simulink model "Shin_com"  (R2024a)
settings: Solver=VariableStepAuto  StartTime=0.0  StopTime=10.0  RelTol=1e-3
undefined symbols (not defined in the file): route1_waypoint_x, route1_waypoint_y, route2_waypoint_x, route2_waypoint_y, route3_waypoint_x, route3_waypoint_y, route4_waypoint_x, route4_waypoint_y, route5_waypoint_x, route5_waypoint_y
libraries: CarMaker4SL x162, slpidlib x4, robotalgslib x1, matrix_library x1
(part 4 of 4)

== matlab function Shin_com/Triggered Subsystem2/Function-Call Subsystem/MATLAB Function4 ==
  data: start input; goal input; obstacle_list input; full_path output
function full_path = main_rrt_rs(start, goal, obstacle_list) %#codegen

    space = [0, 100, -100, 0];
    max_iter = 3000; step_size = 1; goal_sample_rate = 0.4; radius = 10; R = 7;
    MAX_NODES = 3000;
    default_node = struct('pos', zeros(1,3), 'parent', int32(0), 'cost', Inf);
    nodes = repmat(default_node, 1, MAX_NODES);
    nodes(1).pos = start(:)';
    nodes(1).parent = int32(0);
    nodes(1).cost = 0.0;
    node_count = int32(1);
    goal = reshape(goal, 1, 3);
    start = reshape(start, 1, 3);

    c_best = inf; best_goal_node = int32(-1);
    rs_to_goal = NaN(200,3); rs_count = int32(0);

    for iter = 1:max_iter
        if rand < goal_sample_rate
            sample = goal;
        elseif isfinite(c_best)
            sample = informed_sample(start, goal, c_best, space);
        else
            sample = [ ...
                rand_range(space(1), space(2)), ...
                rand_range(space(3), space(4)), ...
                rand * 2 * pi ...
                ];
        end
        sample = reshape(sample, 1, 3);  % ✅ 안전성 확보
        min_dist = inf;
        nearest_id = int32(1);
        for i = 1:node_count
            d = norm(nodes(i).pos(1:2) - sample(1:2));
            if d < min_dist
                min_dist = d;
                nearest_id = int32(i);
            end
        end
        nearest_node = nodes(nearest_id);

        theta = atan2(sample(2) - nearest_node.pos(2), sample(1) - nearest_node.pos(1));
        new_pos = [nearest_node.pos(1:2) + step_size * [cos(theta), sin(theta)], theta];

        if ~collision_check_line(nearest_node.pos, new_pos, obstacle_list, space)
            new_node = struct('pos', new_pos, ...
                'parent', int32(nearest_id), ...
                'cost', nearest_node.cost + norm(new_pos(1:2) - nearest_node.pos(1:2)));

            for i = 1:node_count
                if norm(nodes(i).pos(1:2) - new_node.pos(1:2)) < radius
                    temp_cost = nodes(i).cost + norm(nodes(i).pos(1:2) - new_node.pos(1:2));
                    if temp_cost < new_node.cost && ~collision_check_line(nodes(i).pos, new_node.pos, obstacle_list, space)
                        new_node.cost = temp_cost;
                        new_node.parent = int32(i);
                    end
                end
            end

            if node_count < MAX_NODES
                node_count = node_count + 1;
                nodes(node_count) = new_node;
            end

            if norm(new_node.pos(1:2) - goal(1:2)) < 25
                [valid, rs_path] = reeds_shepp_connect(new_node.pos, goal, R, obstacle_list, space);
                if valid
                    c_rs = new_node.cost + compute_rs_cost(rs_path);
                    if c_rs < c_best
                        c_best = c_rs;
                        best_goal_node = node_count;
                        rs_count = int32(min(size(rs_path,1), size(rs_to_goal,1)));
                        rs_to_goal(1:rs_count,:) = rs_path(1:rs_count,:);
                    end
                end
            end
        end
    end

    if best_goal_node > 0
        path_temp = zeros(300, 3);
        count = int32(0);
        current = best_goal_node;
        while current > 0
            count = count + 1;
            path_temp(count,:) = nodes(current).pos;
            current = nodes(current).parent;
        end
        rrt_path = flipud(path_temp(1:count,:));
        rrt_path = path_clothoid_smoothing(rrt_path); % 고급 smoothing 적용
        n_rrt = size(rrt_path,1);
        full_path = NaN(300,3);
        full_path(1:n_rrt,:) = rrt_path;
        full_path(n_rrt+1:n_rrt+rs_count,:) = rs_to_goal(1:rs_count,:);
    else
        full_path = NaN(300,3);
    end
    function r = rand_range(a, b) %#codegen
        r = a + (b - a) * rand;
    end
end
function sample = informed_sample(start, goal, c_max, space) %#codegen
    % === 고정된 출력: 반드시 [1×3] 벡터 ===
    sample = zeros(1, 3);

    % === 타원 파라미터 계산 ===
    c_min = norm(goal(1:2) - start(1:2));
    a = c_max / 2;
    b = sqrt(max(1e-6, c_max^2 - c_min^2)) / 2;
    theta = atan2(goal(2) - start(2), goal(1) - start(1));
    cos_t = cos(theta);
    sin_t = sin(theta);
    mid = 0.5 * (start(1:2) + goal(1:2));

    % === 고정 반복 횟수 시도 (예: 50회) ===
    for i = 1:50
        x = a * (2 * rand - 1);  % [-a, a]
        y = b * (2 * rand - 1);  % [-b, b]

        % 타원 내부 점만 사용
        if (x^2 / a^2 + y^2 / b^2) <= 1
            pos_x = cos_t * x - sin_t * y + mid(1);
            pos_y = sin_t * x + cos_t * y + mid(2);
            yaw   = 2 * pi * rand;

            sample(1) = pos_x;
            sample(2) = pos_y;
            sample(3) = yaw;
            return;
        end
    end

    % 실패 시 fallback: goal 반환
    sample = goal(:)';  % [1×3] 형태 유지
end

function smooth_path = path_clothoid_smoothing(path)
    if size(path, 1) < 3
        smooth_path = path;
        return;
    end

    fixed_points = false(size(path, 1), 1);
    for i = 2:size(path, 1) - 1
        prev = path(i - 1, 1:2);
        curr = path(i, 1:2);
        next = path(i + 1, 1:2);
        angle1 = atan2(curr(2) - prev(2), curr(1) - prev(1));
        angle2 = atan2(next(2) - curr(2), next(1) - curr(1));
        if abs(angle1 - angle2) < deg2rad(5)
            fixed_points(i) = true;
        end
    end

    x = path(:, 1); y = path(:, 2); yaw = path(:, 3);
    s = cumsum([0; sqrt(diff(x).^2 + diff(y).^2)]);
    ts = linspace(0, s(end), 5 * numel(s));
    x_smooth = interp1(s(~fixed_points), x(~fixed_points), ts, 'pchip', 'extrap');
    y_smooth = interp1(s(~fixed_points), y(~fixed_points), ts, 'pchip', 'extrap');
    yaw_unwrap = unwrap(yaw);
    yaw_smooth = interp1(s(~fixed_points), yaw_unwrap(~fixed_points), ts, 'pchip', 'extrap');

    dx = gradient(x_smooth); dy = gradient(y_smooth);
    ddx = gradient(dx); ddy = gradient(dy);
    curvature = abs((dx .* ddy - dy .* ddx) ./ (dx.^2 + dy.^2).^(3/2));
    max_curvature = 0.05;

    for k = 2:length(curvature)
        if curvature(k) > max_curvature
            factor = max_curvature / curvature(k);
            x_smooth(k) = x_smooth(k-1) + factor * (x_smooth(k) - x_smooth(k-1));
            y_smooth(k) = y_smooth(k-1) + factor * (y_smooth(k) - y_smooth(k-1));
        end
    end
    smooth_path = [x_smooth',...
                    y_smooth',...
                    wrapToPi(yaw_smooth')];
end

function [valid, rs_path] = reeds_shepp_connect(start, goal, R, obstacle_list, space)
    param.step = 0.5;
    param.max_curv = 1 / R;
    [x_list, y_list, yaw_list] = generation(start, goal, param);
    rs_path = [x_list(:), y_list(:), yaw_list(:)];
    valid = true;
    for i = 1:size(rs_path,1)
        pos = rs_path(i, :);
        if collision_check_point(pos, obstacle_list, space)
            valid = false;
            return;
        end
    end
end

function cost = compute_rs_cost(rs_path)
    % rs_path: [N x 3] 형태의 Reeds-Shepp 경로 (x, y, yaw)
    % 두 점 사이의 유클리디안 거리 누적합을 사용한 비용 계산
    if size(rs_path,1) < 2
        cost = 0;
        return;
    end
    dx = diff(rs_path(:,1));
    dy = diff(rs_path(:,2));
    dist = hypot(dx, dy);
    cost = sum(dist);
end

function is_collision = collision_check_line(start_pos, end_pos, obstacle_list, space) %#codegen
    % 간단한 선분-장애물 교차 검사: 샘플링 방식 사용
    n = 10;
    is_collision = false;
    for i = 0:n
        t = i / n;
        pos = (1 - t) * start_pos + t * end_pos;
        if collision_check_point(pos, obstacle_list, space)
            is_collision = true;
            return;
        end
    end
end

function is_collision = collision_check_point(pos, obstacle_list, space)
    x = pos(1); y = pos(2);
    if x < space(1) || x > space(2) || y < space(3) || y > space(4)
        is_collision = true;
        return;
    end
    is_collision = false;
    for i = 1:size(obstacle_list, 1)
        dx = x - obstacle_list(i,1);
        dy = y - obstacle_list(i,2);
        if hypot(dx, dy) < obstacle_list(i,3) + 1.5
            is_collision = true;
            return;
        end
    end
end

function [x_list, y_list, yaw_list] = generation(start_pose, goal_pose, param)
    sx = start_pose(1); sy = start_pose(2); syaw = start_pose(3);
    gx = goal_pose(1); gy = goal_pose(2); gyaw = goal_pose(3);

    dx = gx - sx; dy = gy - sy; dyaw = gyaw - syaw;
    x = (cos(syaw) * dx + sin(syaw) * dy) * param.max_curv;
    y = (-sin(syaw) * dx + cos(syaw) * dy) * param.max_curv;
    planner_fns = {@SCS, @CCC, @CSC, @CCCC, @CCSC};

    best_cost = inf;
    best_path = struct('segs', zeros(1,3), 'ctypes', ['L','S','L'], 'len', inf);

    % === 3) 각 플래너로부터 후보 경로 받아 최저 비용 갱신 ===
    for pi = 1:numel(planner_fns)
        paths = planner_fns{pi}(x, y, dyaw);
        for k = 1:numel(paths)
            if paths(k).len < best_cost
                best_cost = paths(k).len;
                best_path = paths(k);
            end
        end
    end

    % === 4) 유효한 경로가 하나도 없으면 빈 배열 리턴(선택사항) ===
    if isinf(best_cost)
        x_list = zeros(0,1); 
        y_list = zeros(0,1); 
        yaw_list = zeros(0,1);
        return;
    end

    points_num = floor(best_cost / param.step) + length(best_path.segs) + 5;
    x_list_ = zeros(points_num, 1);
    y_list_ = zeros(points_num, 1);
    yaw_list_ = zeros(points_num, 1);

    i = 1;
    x = 0; y = 0; yaw = 0;
    for j = 1:length(best_path.segs)
        m = best_path.ctypes(j);
        seg_length = best_path.segs(j);
        if seg_length == 0
            continue;   % 0 길이 세그먼트는 건너뛸 것
        end
        d_length = param.step * sign(seg_length);
        l = 0;
        while abs(l) <= abs(seg_length)
            new_pt = interpolate(m, l, [x, y, yaw], param);
            i = i + 1;
            x_list_(i) = new_pt(1);
            y_list_(i) = new_pt(2);
            yaw_list_(i) = new_pt(3);
            l = l + d_length;
        end
        new_pt = interpolate(m, seg_length, [x, y, yaw], param);
        i = i + 1;
        x_list_(i) = new_pt(1);
        y_list_(i) = new_pt(2);
        yaw_list_(i) = new_pt(3);
        x = new_pt(1); y = new_pt(2); yaw = new_pt(3);
    end

    x_list_ = x_list_(1:i);
    y_list_ = y_list_(1:i);
    yaw_list_ = yaw_list_(1:i);

    x_list = zeros(size(x_list_));
    y_list = zeros(size(y_list_));
    yaw_list = zeros(size(yaw_list_));
    for k = 1:length(x_list_)
        x_list(k) = cos(-syaw) * x_list_(k) + sin(-syaw) * y_list_(k) + sx;
        y_list(k) = -sin(-syaw) * x_list_(k) + cos(-syaw) * y_list_(k) + sy;
        yaw_list(k) = M(yaw_list_(k) + syaw);
    end
end

function [r, theta] = R(x, y)
    r = hypot(x, y);
    theta = atan2(y, x);
end

function theta_truncate = M(theta)
    while theta > pi
        theta = theta - 2.0 * pi;
    end
    while theta < -pi
        theta = theta + 2.0 * pi;
    end
    theta_truncate = theta;
end

function [tau, omega] = calTauOmega(u, v, xi, eta, phi)
    delta = M(u - v);
    A = sin(u) - sin(delta);
    B = cos(u) - cos(delta) - 1.0;

    t1 = atan2(eta * A - xi * B, xi * A + eta * B);
    t2 = 2.0 * (cos(delta) - cos(v) - cos(u)) + 3.0;

    if t2 < 0
        tau = M(t1 + pi);
    else
        tau = M(t1);
    end
    omega = M(tau - u + v - phi);
end
function segs = SLS(x, y, phi)
    % Straight-Left-Straight generation mode.
    segs = [];
    
    phi = M(phi);
    if y > 0.0 && phi > 0.0 && phi < pi * 0.99
        xd = -y / tan(phi) + x;
        t = xd - tan(phi / 2.0);
        u = phi;
        v = hypot(x - xd, y) - tan(phi / 2.0);
        segs = [t, u, v];
    elseif y < 0.0 && phi > 0.0 && phi < pi * 0.99
        xd = -y / tan(phi) + x;
        t = xd - tan(phi / 2.0);
        u = phi;
        v = -hypot(x - xd, y) - tan(phi / 2.0);
        segs = [t, u, v];
    end
end

function segs = LRL(x, y, phi)
    % Left-Right-Left generation mode. (L+R-L-)
    segs = [];
    [r, theta] = R(x - sin(phi), y - 1.0 + cos(phi));
    if r <= 4.0
        u = -2.0 * asin(0.25 * r);
        t = M(theta + 0.5 * u + pi);
        v = M(phi - t + u);
        if t >= 0.0 && u <= 0.0
            segs = [t, u, v];
        end
    end
end

function segs = LSL(x, y, phi)
    % Left-Straight-Left generation mode. (L+S+L+)
    segs = [];
    
    [u, t] = R(x - sin(phi), y - 1.0 + cos(phi));
    if t >= 0.0
        v = M(phi - t);
        if v >= 0.0
            segs = [t, u, v];
        end
    end
end

function segs = LSR(x, y, phi)
    % Left-Straight-Right generation mode. (L+S+R+)
    segs = [];
    
    [r, theta] = R(x + sin(phi), y - 1.0 - cos(phi));
    r = r * r;
    if r >= 4.0
        u = sqrt(r - 4.0);
        t = M(theta + atan2(2.0, u));
        v = M(t - phi);
        if t >= 0.0 && v >= 0.0
            segs = [t, u, v];
        end
    end
end

function segs = LRLRn(x, y, phi)
    % Left-Right(beta)-Left(beta)-Right generation mode. (L+R+L-R-)
    segs = [];
    
    xi = x + sin(phi);
    eta = y - 1.0 - cos(phi);
    rho = 0.25 * (2.0 + hypot(xi, eta));
    if rho <= 1.0
        u = acos(rho);
        [t, v] = calTauOmega(u, -u, xi, eta, phi);
        if t >= 0.0 && v <= 0.0
            segs = [t, u, v];
        end
    end
end

function segs = LRLRp(x, y, phi)
    % Left-Right(beta)-Left(beta)-Right generation mode. (L+R-L-R+)
    segs = [];
    
    xi = x + sin(phi);
    eta = y - 1.0 - cos(phi);
    rho = (20.0 - xi * xi - eta * eta) / 16.0;
    if 0.0 <= rho && rho <= 1.0
        u = -acos(rho);
        if u >= -0.5 * pi
            [t, v] = calTauOmega(u, u, xi, eta, phi);
            if t >= 0.0 && v >= 0.0
                segs = [t, u, v];
            end
        end
    end
end

function segs = LRSR(x, y, phi)
    % Left-Right(pi/2)-Straight-Right generation mode. (L+R-S-R-)
    segs = [];
    
    xi = x + sin(phi);
    eta = y - 1.0 - cos(phi);
    [rho, theta] = R(-eta, xi);

    if rho >= 2.0
        t = theta;
        u = 2.0 - rho;
        v = M(t + 0.5 * pi - phi);
        if t >= 0.0 && u <= 0.0 && v <= 0.0
            segs = [t, u, v];
        end
    end
end

function segs = LRSL(x, y, phi)
    % Left-Right(pi/2)-Straight-Left generation mode. (L+R-S-L-)
    segs = [];
    
    xi = x - sin(phi);
    eta = y - 1.0 + cos(phi);
    [rho, theta] = R(xi, eta);
    if rho >= 2.0
        r = sqrt(rho * rho - 4.0);
        u = 2.0 - r;
        t = M(theta + atan2(r, -2.0));
        v = M(phi - 0.5 * pi - t);
        if t >= 0.0 && u <= 0.0 && v <= 0.0
            segs = [t, u, v];
        end
    end
end

function segs = LRSLR(x, y, phi)
    % Left-Right(pi/2)-Straight-Left(pi/2)-Right generation mode. (L+R-S-L-R+)
    segs = [];
    
    xi = x + sin(phi);
    eta = y - 1.0 - cos(phi);
    [r, ~] = R(xi, eta);
    if r >= 2.0
        u = 4.0 - sqrt(r * r - 4.0);
        if u <= 0.0
            t = M(atan2((4.0 - u) * xi - 2.0 * eta, -2.0 * xi + (u - 4.0) * eta));
            v = M(t - phi);
            if t >= 0.0 && v >= 0.0
                segs = [t, u, v];
            end
        end
    end
end

function path = RSPath(segs_in, ctypes_in)
    MAX_LEN = 5;  % 최대 5개 segment까지 허용
    segs_fixed = zeros(1, MAX_LEN);
    ctypes_fixed = repmat(' ', 1, MAX_LEN);

    n = length(segs_in);
    segs_fixed(1:n) = segs_in;

    for i = 1:n
        ctypes_fixed(i) = ctypes_in{i};
    end

    path.segs = segs_fixed;
    path.ctypes = ctypes_fixed;
    path.len = sum(abs(segs_in(:)));  % ✅ 항상 스칼라
end

    
function paths = SCS(x, y, phi) %#codegen
    MAX_PATHS = 2;
    paths = init_rs_paths(MAX_PATHS);
    cnt = uint8(0);

    segs = SLS(x, y, phi);
    if ~isempty(segs)
        cnt = cnt + 1;
        paths(cnt) = RSPath(segs, {'S', 'L', 'S'});
    end

    segs = SLS(x, -y, -phi);
    if ~isempty(segs)
        cnt = cnt + 1;
        paths(cnt) = RSPath(segs, {'S', 'R', 'S'});
    end

    paths = paths(1:cnt);
end

function paths = CCC(x, y, phi) %#codegen
    MAX_PATHS = 8;
    paths = init_rs_paths(MAX_PATHS);
    cnt = uint8(0);

    cases = {
        LRL(x, y, phi),            {'L','R','L'};
        -LRL(-x, y, -phi),         {'L','R','L'};
        LRL(x, -y, -phi),          {'R','L','R'};
        -LRL(-x, -y, phi),         {'R','L','R'};
    };

    for k = 1:size(cases,1)
        segs = cases{k,1};
        if ~isempty(segs)
            cnt = cnt + 1;
            paths(cnt) = RSPath(segs, cases{k,2});
        end
    end

    xb = x * cos(phi) + y * sin(phi);
    yb = x * sin(phi) - y * cos(phi);

    segs = LRL(xb, yb, phi);
    if ~isempty(segs)
        cnt = cnt + 1;
        paths(cnt) = RSPath([segs(3), segs(2), segs(1)], {'L','R','L'});
    end

    segs = LRL(-xb, yb, -phi);
    if ~isempty(segs)
        cnt = cnt + 1;
        paths(cnt) = RSPath(-[segs(3), segs(2), segs(1)], {'L','R','L'});
    end

    segs = LRL(xb, -yb, -phi);
    if ~isempty(segs)
        cnt = cnt + 1;
        paths(cnt) = RSPath([segs(3), segs(2), segs(1)], {'R','L','R'});
    end

    segs = LRL(-xb, -yb, phi);
    if ~isempty(segs)
        cnt = cnt + 1;
        paths(cnt) = RSPath(-[segs(3), segs(2), segs(1)], {'R','L','R'});
    end

    paths = paths(1:cnt);
end

function paths = CSC(x, y, phi) %#codegen
    MAX_PATHS = 8;
    paths = init_rs_paths(MAX_PATHS);
    cnt = uint8(0);

    segs_and_types = {
        LSL(x, y, phi),            {'L', 'S', 'L'};
        -LSL(-x, y, -phi),         {'L', 'S', 'L'};
        LSL(x, -y, -phi),          {'R', 'S', 'R'};
        -LSL(-x, -y, phi),         {'R', 'S', 'R'};
        LSR(x, y, phi),            {'L', 'S', 'R'};
        -LSR(-x, y, -phi),         {'L', 'S', 'R'};
        LSR(x, -y, -phi),          {'R', 'S', 'L'};
        -LSR(-x, -y, phi),         {'R', 'S', 'L'};
    };

    for k = 1:size(segs_and_types, 1)
        segs = segs_and_types{k,1};
        if ~isempty(segs)
            cnt = cnt + 1;
            paths(cnt) = RSPath(segs, segs_and_types{k,2});
        end
    end

    paths = paths(1:cnt);
end

function paths = CCCC(x, y, phi) %#codegen
    MAX_PATHS = 8;
    paths = init_rs_paths(MAX_PATHS);
    cnt = uint8(0);

    segs = LRLRn(x, y, phi);
    if ~isempty(segs)
        cnt = cnt + 1;
        paths(cnt) = RSPath([segs(1), segs(2), -segs(2), segs(3)], {'L','R','L','R'});
    end

    segs = LRLRn(-x, y, -phi);
    if ~isempty(segs)
        cnt = cnt + 1;
        paths(cnt) = RSPath([-segs(1), -segs(2), segs(2), -segs(3)], {'L','R','L','R'});
    end

    segs = LRLRn(x, -y, -phi);
    if ~isempty(segs)
        cnt = cnt + 1;
        paths(cnt) = RSPath([segs(1), segs(2), -segs(2), segs(3)], {'R','L','R','L'});
    end

    segs = LRLRn(-x, -y, phi);
    if ~isempty(segs)
        cnt = cnt + 1;
        paths(cnt) = RSPath([-segs(1), -segs(2), segs(2), -segs(3)], {'R','L','R','L'});
    end

    segs = LRLRp(x, y, phi);
    if ~isempty(segs)
        cnt = cnt + 1;
        paths(cnt) = RSPath([segs(1), segs(2), segs(2), segs(3)], {'L','R','L','R'});
    end

    segs = LRLRp(-x, y, -phi);
    if ~isempty(segs)
        cnt = cnt + 1;
        paths(cnt) = RSPath([-segs(1), -segs(2), -segs(2), -segs(3)], {'L','R','L','R'});
    end

    segs = LRLRp(x, -y, -phi);
    if ~isempty(segs)
        cnt = cnt + 1;
        paths(cnt) = RSPath([segs(1), segs(2), segs(2), segs(3)], {'R','L','R','L'});
    end

    segs = LRLRp(-x, -y, phi);
    if ~isempty(segs)
        cnt = cnt + 1;
        paths(cnt) = RSPath([-segs(1), -segs(2), -segs(2), -segs(3)], {'R','L','R','L'});
    end

    paths = paths(1:cnt);
end

function paths = CCSC(x, y, phi) %#codegen
    MAX_PATHS = 16;
    paths = init_rs_paths(MAX_PATHS);
    cnt = uint8(0);

    variants = {
        LRSL(x, y, phi),           {'L', 'R', 'S', 'L'}, [1 -0.5*pi 2 3];
        LRSL(-x, y, -phi),         {'L', 'R', 'S', 'L'}, [-1 0.5*pi -2 -3];
        LRSL(x, -y, -phi),         {'R', 'L', 'S', 'R'}, [1 -0.5*pi 2 3];
        LRSL(-x, -y, phi),         {'R', 'L', 'S', 'R'}, [-1 0.5*pi -2 -3];
        LRSR(x, y, phi),           {'L', 'R', 'S', 'R'}, [1 -0.5*pi 2 3];
        LRSR(-x, y, -phi),         {'L', 'R', 'S', 'R'}, [-1 0.5*pi -2 -3];
        LRSR(x, -y, -phi),         {'R', 'L', 'S', 'L'}, [1 -0.5*pi 2 3];
        LRSR(-x, -y, phi),         {'R', 'L', 'S', 'L'}, [-1 0.5*pi -2 -3];
    };

    for k = 1:size(variants,1)
        segs = variants{k,1};
        type = variants{k,2};
        idxs = variants{k,3};
        if ~isempty(segs)
            t = segs(abs(idxs(1))) * sign(idxs(1));
            u = segs(abs(idxs(3))) * sign(idxs(3));
            v = segs(abs(idxs(4))) * sign(idxs(4));
            paths(cnt + 1) = RSPath([t, idxs(2), u, v], type);
            cnt = cnt + 1;
        end
    end

    paths = paths(1:cnt);
end

function out = init_rs_paths(N)
    tmpl = struct('segs', zeros(1,5), 'ctypes', repmat(' ',1,5), 'len', 0);
    out = repmat(tmpl, N, 1);
end

function new_pt = interpolate(mode, length, init_pose, param)
    x = init_pose(1); y = init_pose(2); yaw = init_pose(3);

    if mode == 'S'
        new_x   = x + length / param.max_curv * cos(yaw);
        new_y   = y + length / param.max_curv * sin(yaw);
        new_yaw = yaw;
    elseif mode == 'L'
        new_x   = x + (sin(yaw + length) - sin(yaw)) / param.max_curv;
        new_y   = y - (cos(yaw + length) - cos(yaw)) / param.max_curv;
        new_yaw = yaw + length;
    elseif mode == 'R'
        new_x   = x - (sin(yaw - length) - sin(yaw)) / param.max_curv;
        new_y   = y + (cos(yaw - length) - cos(yaw)) / param.max_curv;
        new_yaw = yaw - length;
    else
        new_x = 0; new_y = 0; new_yaw = 0;
    end
    new_pt = [new_x, new_y, new_yaw];
end

== matlab function Shin_com/Triggered Subsystem2/Function-Call Subsystem1/MATLAB Function ==
  data: currPoseRear input; v input; waypoints input; delta output
function delta = lateral_spp_controller(currPoseRear, v, waypoints)
%▴ Hybrid Stanley & Pure Pursuit + Monotonic Index Enforcement
% Inputs:
%   currPoseRear : [x_rear; y_rear; psi] (후륜축 기준 위치 및 자세)
%   v            : 현재 속도 (m/s)
%   waypoints    : N×3 [x_i, y_i, psi_i] (경로 웨이포인트)
% Output:
%   delta        : 전륜 조향각 (rad)

    %#codegen
    %% persistent 변수 초기화
    persistent idx_last delta_prev
    if isempty(idx_last)
        idx_last   = 1;    % 마지막 타겟 인덱스 (초기값)
    end
    if isempty(delta_prev)
        delta_prev = 0;    % 이전 조향각 (로우패스 필터용)
    end

    %% 파라미터
    L        = 2.9;                             % 휠베이스 [m]
    k_st     = 1.0;                             % Stanley 이득
    eps_v    = 0.1;                             % 속도 안정화 상수
    deltaMax = deg2rad(40);                     % 최대 조향각 제한 ±40°
    e_thresh = 0.5;                             % SPP 전환 임계값 [m]
    k_pp     = 0.3;                             % 룩어헤드 속도 이득
    Ld_min   = 2.0;                             % 룩어헤드 최솟값 [m]
    Ld_max   = 4.0;                             % 룩어헤드 최댓값 [m]
    alpha_f  = 0.35;                            % 로우패스 필터 상수

    %% 전륜축 위치 계산 (후륜축 기준 → 전륜축 좌표 변환)
    x_f = currPoseRear(1) + L*cos(currPoseRear(3));
    y_f = currPoseRear(2) + L*sin(currPoseRear(3));

    %% 전방 웨이포인트만 선별 (로컬 좌표계)
    psi_wrapped = wrapToPi(currPoseRear(3));    % yaw를 –π~π로 유지
    heading_vec = [cos(psi_wrapped), sin(psi_wrapped)];
    diffs       = waypoints(:,1:2) - currPoseRear(1:2)';
    forward_idx = find(diffs * heading_vec' > 0);  % 전방 idx
    if isempty(forward_idx)
        forward_idx = (1:size(waypoints,1))';       % 전방이 없으면 전체 사용
    end

    %% 룩어헤드 거리 계산
    Ld_raw = k_pp * v + eps_v;
    Ld     = min(max(Ld_raw, Ld_min), Ld_max);

    %% 후보 인덱스 범위 설정 (룩어헤드 윈도우)
    N = size(waypoints,1);
    extra     = round(0.2 * Ld);                  % 윈도우 여분
    start_idx = max(idx_last - extra, 1);
    end_idx   = min(idx_last + round(Ld) + extra, N);
    cand_idx  = intersect(forward_idx, (start_idx:end_idx)');

    if isempty(cand_idx)
        cand_idx = forward_idx;  % 후보 없으면 전방 전체 사용
    end

    %% 최단거리 웨이포인트 선택
    dists = hypot(waypoints(cand_idx,1)-x_f, waypoints(cand_idx,2)-y_f);
    [~, rel] = min(dists);
    idx_new  = cand_idx(rel);  % 새로 계산된 인덱스

    %% 1) Monotonic Index Enforcement 적용
    % 새 인덱스(idx_new)가 이전 idx_last보다 작으면 무시
    if idx_new < idx_last
        idx_last = idx_last;    % 변경 없이 유지
    else
        idx_last = idx_new;     % 증가 시에만 갱신
    end

    %% 참조점 정보 추출
    x_ref   = waypoints(idx_last,1);
    y_ref   = waypoints(idx_last,2);
    psi_ref = waypoints(idx_last,3);

    %% Heading error 및 Cross-Track error 계산
    theta_e = wrapToPi(psi_ref - currPoseRear(3));  
    e_cte   = -(x_f - x_ref)*sin(psi_ref) + (y_f - y_ref)*cos(psi_ref);

    %% 제어 분기: Pure Pursuit vs Stanley
    if abs(e_cte) > e_thresh
        % Pure Pursuit
        alpha     = wrapToPi(atan2(y_ref-currPoseRear(2), x_ref-currPoseRear(1)) ...
                     - currPoseRear(3));
        delta_cmd = atan2(2 * L * sin(alpha), Ld);
    else
        % Stanley
        delta_cmd = theta_e + atan((k_st * e_cte) / (v + eps_v));
    end

    %% 로우패스 필터 적용 및 조향각 포화
    delta       = alpha_f * delta_cmd + (1 - alpha_f) * delta_prev;
    delta_prev  = delta;  
    delta       = max(min(delta, deltaMax), -deltaMax);

end

== matlab function Shin_com/Triggered Subsystem2/Function-Call Subsystem1/MATLAB Function2 ==
  settings: sampleTime=0.05
  data: currPoseRear input; DesiredAx output; ego_v input; target_velocity input; goalPose input; stopFlag output; target_velocity output
function [DesiredAx,stopFlag,target_velocity] = longitudinal_goal_controller(currPoseRear, ego_v,target_velocity,goalPose)
%▴ 종방향 속도 제어 및 목표 도달 확인
% Inputs:
%   currPoseRear: [x_rear; y_rear; psi] (후륜축 기준)
%   v           : 속도 (m/s)
%   goalPose    : [x_goal; y_goal; psi_goal]
% Outputs:
%   DesiredAx   : 원하는 가속도 (m/s^2)
%   stopFlag    : 목표 도달 시 true

    persistent Kp Kd dt prev_error
  if isempty(Kp)
    % — PD 게인 설정 (필요에 따라 조정하세요) —
    Kp = 1.8;    % 비례 이득
    Kd = 0.1;    % 미분 이득
    % — 제어 업데이트 주기 (Simulink 샘플타임과 동일하게) —
    dt = 0.1;    % [s]
    % — previous error 초기화 —
    prev_error = target_velocity - ego_v;
  end

  % 1) 속도 오차
  error = target_velocity - ego_v;
  % 2) 오차 변화율 (미분항)
  derivative = (error - prev_error) / dt;
  % 3) PD 제어 법칙
  DesiredAx = Kp * error + Kd * derivative;
  % 4) 이전 오차 갱신
  prev_error = error;


    %#codegen
    % 1) 위치·헤딩 오차 계산
    dx     = currPoseRear(1) - goalPose(1);
    dy     = currPoseRear(2) - goalPose(2);
    dist   = hypot(dx, dy);                                           % 거리 계산 :contentReference[oaicite:3]{index=3}
    yawErr = wrapToPi(goalPose(3) - currPoseRear(3));                 % –π~π 범위 :contentReference[oaicite:4]{index=4}

    % 2) 목표 도달 여부 판단 (Goal Checking in Parking Valet) :contentReference[oaicite:5]{index=5}
    posTol = 1.7;             % 위치 허용 오차 [m]
    yawTol = deg2rad(30);     % 헤딩 허용 오차 [rad]
    almostFlag = dist<12;
    distFlag = dist <= posTol;
    yawFlag = abs(yawErr) <= yawTol
    stopFlag = distFlag && yawFlag;

    % 3) DesiredAx 계산
    if stopFlag
        DesiredAx = -1000;
        disp("stopFlag")% 도착 시 완전 정지
    elseif almostFlag
        target_velocity = 3;
        disp("almost goal")% 근접 시 제동 가속도
        error      = target_velocity - ego_v;
        derivative = (error - prev_error)/dt;
        DesiredAx  = Kp*error + Kd*derivative;
        prev_error = error;
    end
end

== matlab function Shin_com/Triggered Subsystem2/Function-Call Subsystem1/MATLAB Function4 ==
  settings: sampleTime=0.05
  data: poly_coeff input; lateral_error output; velocity input; lookahead_time input; x_lookahead output
function [lateral_error, x_lookahead] = compute_lateral_error(poly_coeff, velocity, lookahead_time)
    
    % Lookahead 지점 계산
    x_lookahead = velocity * lookahead_time;
    % 경로 상의 lookahead 지점에서의 y값 계산
    y_desired = polyval(poly_coeff, x_lookahead);

    % lateral error : 차량 y=0 위치와 경로 y_desired의 차이
    lateral_error = y_desired;
end

== matlab function Shin_com/Triggered Subsystem2/Function-Call Subsystem1/MATLAB Function4  ==
  settings: sampleTime=0.05
  data: path input; local_waypoints_ output; vehicle_position input; head input
function local_waypoints_ = global_to_local_waypoints(path, vehicle_position, head)
    %#codegen
    % 글로벌 경로를 로컬 경로로 변환해주는 함수
    % path : [x, y, yaw] (경로 점들)
    % vehicle_position : [Ego_Global_X, Ego_Global_Y]
    % head : Ego_Yaw (rad)
    % 출력: 로컬 좌표 (x_local, y_local, yaw_local)

    % 최대 경로 점 개수 설정
    max_points = 100;

    % 초기화
    local_waypoints_ = NaN(max_points, 3);  % 고정 크기 배열

    % 차량 위치 및 헤딩 추출
    ego_x = vehicle_position(1);
    ego_y = vehicle_position(2);
    ego_yaw = head;

    % 회전 행렬 생성 (글로벌→로컬 변환)
    R = [cos(-ego_yaw) -sin(-ego_yaw); 
         sin(-ego_yaw)  cos(-ego_yaw)];

    count = int32(0);  % 경로 점 개수

    % 각 경로 포인트에 대해 변환 수행
    for i = 1:min(size(path, 1), max_points)
        % 글로벌 좌표에서 차량까지의 상대 위치
        dx = path(i, 1) - ego_x;  % X 좌표 차이
        dy = path(i, 2) - ego_y;  % Y 좌표 차이

        % 회전 변환 적용
        local_pos = R * [dx; dy];
        
        % Yaw 변환: 로컬 좌표계에서의 Yaw
        global_yaw = path(i, 3);
        local_yaw = wrapToPi(global_yaw - ego_yaw);  % 로컬 yaw 변환

        % 차량으로부터 waypoint까지의 거리
        distance = sqrt(local_pos(1)^2 + local_pos(2)^2);

        % 첫 번째 유효 경로 점 저장 (x > 0인 첫 포인트)
        if count == 0 && local_pos(1) > 0
            count = count + 1;
            local_waypoints_(count, :) = [local_pos(1), local_pos(2), local_yaw];
        end
        
        % 고정 크기 초과 방지
        if count < max_points
            count = count + 1;
            local_waypoints_(count, :) = [local_pos(1), local_pos(2), local_yaw];
        else
            warning('Maximum number of waypoints reached.');
            break;
        end
    end

    % 남은 부분을 NaN으로 채움
    if count < max_points
        local_waypoints_((count+1):max_points, :) = NaN;
    end
end

== matlab function Shin_com/Triggered Subsystem2/Function-Call Subsystem1/MATLAB Function5 ==
  settings: sampleTime=0.05
  data: local_waypoints input; poly_coeff output
function poly_coeff = fit_polynomial_to_waypoints(local_waypoints)
    % waypoint를 curve fitting 한 다항식 계수 반환
    % input: 로컬 좌표 웨이포인트
    % output: 다항식 계수 (3차)

    % 웨이포인트 추출
    x_points = local_waypoints(:, 1);  % 로컬 x 좌표
    y_points = local_waypoints(:, 2);  % 로컬 y 좌표

    % 유효한 웨이포인트만 사용 (x 좌표가 양수인 것만)
    valid_indices = x_points > 0;
    x_valid = x_points(valid_indices);
    y_valid = y_points(valid_indices);

    % 웨이포인트가 충분한지 확인
    if length(x_valid) < 4
        % 웨이포인트가 부족하면 직선 경로 반환
        poly_coeff = [0, 0, 0, 0];  % y = 0 (직선)
    else
        % 3차 다항식 피팅 (y = ax^3 + bx^2 + cx + d)
        poly_coeff = polyfit(x_valid, y_valid, 3);
    end
end

== matlab function Shin_com/Triggered Subsystem/MATLAB Function4 1 ==
  settings: sampleTime=0.05
  data: waypoint_x input; waypoint_y input; local_waypoints_ output; vehicle_position input; head input
function local_waypoints_ = global_to_local_waypoints(waypoint_x, waypoint_y, vehicle_position, head)

    % 초기화
    num_points = size(waypoint_x, 1);
    local_waypoints_ = NaN(num_points, 2);  % [x_local, y_local]

    % 차량 위치 추출
    ego_x = vehicle_position(1);
    ego_y = vehicle_position(2);
    ego_yaw = head;

    % 회전 행렬 생성 (글로벌→로컬 변환)
    R = [cos(-ego_yaw) -sin(-ego_yaw); 
         sin(-ego_yaw)  cos(-ego_yaw)];

    count = 0;
    % 각 웨이포인트에 대해 변환 수행
    for i = 1:num_points
        % 글로벌 좌표에서 차량까지의 상대 위치
        dx = waypoint_x(i) - ego_x;  % X 좌표 차이
        dy = waypoint_y(i) - ego_y;  % Y 좌표 차이

        % 회전 변환 적용
        local_pos = R * [dx; dy];
        distance = sqrt(dx.^2 + dy.^2); % 차량으로부터 waypoint까지의 길이 계산

        % 시작 좌표 저장
        if count == 0 && local_pos(1) > 0 && distance < 15
            count = count + 1;
            local_waypoints_(count, :) = [local_pos(1) local_pos(2)];     % 로컬 x 좌표 
        end

        % 아래의 조건을 모두 만족하는 경우에만 좌표 저장
        % 1. x 좌표가 0보다 큰 경우
        % 2. x의 현재 좌표가 이전 x의 좌표보다 큰 경우
        % 3. 차량으로부터 waypoint까지의 길이가 30m 이내인 경우 (길이는 임의로 테스트 한 후 설정 가능할 듯)
        if count  ~= 0 && local_pos(1) > 0 && local_pos(1) > local_waypoints_(count, 1)  && distance < 15
            count = count + 1;
            local_waypoints_(count, :) = [local_pos(1) local_pos(2)];
        end
    end
end

== matlab function Shin_com/Subsystem2/MATLAB Function4 ==
  settings: sampleTime=0.05
  data: poly_coeff input; lateral_error output; velocity input; lookahead_time input; x_lookahead output
function [lateral_error, x_lookahead] = compute_lateral_error(poly_coeff, velocity, lookahead_time)
    % Lookahead 지점 계산
    x_lookahead = velocity * lookahead_time + 2.9;

    % 경로 상의 lookahead 지점에서의 y값 계산
    y_desired = polyval(poly_coeff, x_lookahead);

    % lateral error : 차량 y=0 위치와 경로 y_desired의 차이
    lateral_error = y_desired;
end

== matlab function Shin_com/Subsystem2/MATLAB Function4  ==
  settings: sampleTime=0.05
  data: waypoints input; local_waypoints_ output; vehicle_position input; head input
function local_waypoints_ = global_to_local_waypoints(waypoints, vehicle_position, head)
    % 글로벌 좌표를 로컬 좌표로 변환해주는 함수
    % waypoints : Global_Waypoints [id, X, Y]
    % vehicle_position : [Ego_Global_X, Ego_Global_Y]
    % head : Ego_Yaw (rad)
    % 출력: Local Waypoints

    % 초기화
    num_points = size(waypoints, 1);
    local_waypoints_ = NaN(num_points, 2);  % [x_local, y_local]

    % 차량 위치 추출
    ego_x = vehicle_position(1);
    ego_y = vehicle_position(2);
    ego_yaw = head;

    % 회전 행렬 생성 (글로벌→로컬 변환)
    R = [cos(-ego_yaw) -sin(-ego_yaw); 
         sin(-ego_yaw)  cos(-ego_yaw)];

    count = 0;
    % 각 웨이포인트에 대해 변환 수행
    for i = 1:num_points
        % 글로벌 좌표에서 차량까지의 상대 위치
        dx = waypoints(i, 1) - ego_x;  % X 좌표 차이
        dy = waypoints(i, 2) - ego_y;  % Y 좌표 차이

        % 회전 변환 적용
        local_pos = R * [dx; dy];
        distance = sqrt(dx.^2 + dy.^2); % 차량으로부터 waypoint까지의 길이 계산

        % 시작 좌표 저장
        if count == 0 && local_pos(1) > 0 && distance < 15
            count = count + 1;
            local_waypoints_(count, :) = [local_pos(1) local_pos(2)];     % 로컬 x 좌표 
        end

        % 아래의 조건을 모두 만족하는 경우에만 좌표 저장
        % 1. x 좌표가 0보다 큰 경우
        % 2. x의 현재 좌표가 이전 x의 좌표보다 큰 경우
        % 3. 차량으로부터 waypoint까지의 길이가 30m 이내인 경우 (길이는 임의로 테스트 한 후 설정 가능할 듯)
        if count  ~= 0 && local_pos(1) > 0 && local_pos(1) > local_waypoints_(count, 1)  && distance < 15
            count = count + 1;
            local_waypoints_(count, :) = [local_pos(1) local_pos(2)];
        end
    end
end

== matlab function Shin_com/Subsystem2/MATLAB Function7 ==
  settings: sampleTime=0.05
  data: local_waypoints input; poly_coeff output
function poly_coeff = fit_polynomial_to_waypoints(local_waypoints)
    % waypoint를 curve fitting 한 다항식 계수 반환
    % input: 로컬 좌표 웨이포인트
    % output: 다항식 계수 (3차)

    % 웨이포인트 추출
    x_points = local_waypoints(:, 1);  % 로컬 x 좌표
    y_points = local_waypoints(:, 2);  % 로컬 y 좌표

    % 유효한 웨이포인트만 사용 (x 좌표가 양수인 것만)
    valid_indices = x_points > 0;
    x_valid = x_points(valid_indices);
    y_valid = y_points(valid_indices);
    poly_coeff = polyfit(x_valid, y_valid, 3);
end

== stateflow chart Shin_com/Triggered Subsystem2/Chart1 ==
  settings: sampleTime=0.05
  state drawMap
    entry:
    draw_Map();
  state goParking
    during:
    go_Parking();
  (default) -> drawMap
  drawMap -> goParking : after(10,tick)
  events: go_Parking output FUNCTION_CALL_EVENT; draw_Map output FUNCTION_CALL_EVENT

== matlab function Shin_com/Triggered Subsystem2/Function-Call Subsystem/MATLAB Function ==
  data: path input; ordered_path output
function ordered_path = reorder_path(path)
    %#codegen
    % 입력: path (100x3) - 역순 경로
    % 출력: ordered_path (100x3) - 정순 경로

    % 고정 크기 배열 선언 (100x3)
    ordered_path = NaN(300, 3);  
    
    % 유효 경로 필터링 (NaN 값 제거)
    valid_idx = ~isnan(path(:, 1)) & ~isnan(path(:, 2)) & ~isnan(path(:, 3));
    valid_path = path(valid_idx, :);

    % 유효 경로 개수
    num_points = size(valid_path, 1);

    % 역순으로 배열 채우기 (고정 크기 유지)
    for i = 1:num_points
        ordered_path(i, :) = valid_path(num_points - i + 1, :);
    end

    % 나머지 부분 NaN으로 채우기
    if num_points < 100
        ordered_path((num_points+1):100, :) = NaN;
    end
end

== matlab function Shin_com/Triggered Subsystem/MATLAB Function5 ==
  settings: sampleTime=0.05
  data: x input; x_best output; y input; v input; map_x input; y_best output; map_y input; x_all output; y_all output; obs_x input; obs_y input
function [x_best, y_best, x_all, y_all] = FrenetTrajectoryGenerator(x, y, v, map_x, map_y, obs_x, obs_y)
% 설정
DF_set = [-3.5, 0, 3.5];  % 차선 오프셋 후보 (좌, 중앙, 우)
K_J = 0.1; K_T = 0.1; K_D = 10.0; K_V = 1.0; K_LAT = 2.0; K_LON = 1.0;
target_speed = 15;
T = 1.0;
dt = 0.05;
ego_radius = 2.0;

M = length(DF_set);
N = round(T / dt);

x_all = zeros(N, M);
y_all = zeros(N, M);

% 장애물 정보
obs_r = 2.0;
num_obs = 8;

% 기준 경로 길이 계산
map_s = zeros(length(map_x), 1);
for i = 2:length(map_x)
    dx = map_x(i) - map_x(i-1);
    dy = map_y(i) - map_y(i-1);
    map_s(i) = map_s(i-1) + hypot(dx, dy);
end

% 현재 위치를 Frenet 좌표로 변환
[s0, d0] = getFrenet(x, y, map_x, map_y, map_s);
si = s0; si_d = v; si_dd = 0;
di = d0; di_d = 0; di_dd = 0;

costs = inf(1, M);  % 각 경로의 비용
trajectories = cell(M,2);  % x/y trajectory 저장

for k = 1:M
    d_target = DF_set(k);

    % Lateral (Quintic)
    a0 = di; a1 = di_d; a2 = 0.5 * di_dd;
    A_lat = [T^3 T^4 T^5; 3*T^2 4*T^3 5*T^4; 6*T 12*T^2 20*T^3];
    b_lat = [d_target - a0 - a1*T - a2*T^2; -a1 - 2*a2*T; -2*a2];
    coeff_d = A_lat \ b_lat;

    % Longitudinal (Quartic)
    b0 = si; b1 = si_d; b2 = 0.5 * si_dd;
    A_lon = [3*T^2 4*T^3; 6*T 12*T^2];
    b_lon = [target_speed - b1 - 2*b2*T; -2*b2];
    coeff_s = A_lon \ b_lon;

    s_traj = zeros(N,1); d_traj = zeros(N,1);
    x_traj = zeros(N,1); y_traj = zeros(N,1);
    jerk_d = 0; jerk_s = 0;
    is_collision = false;

    for i = 1:N
        t = (i-1)*dt;
        s_traj(i) = b0 + b1*t + b2*t^2 + coeff_s(1)*t^3 + coeff_s(2)*t^4;
        d_traj(i) = a0 + a1*t + a2*t^2 + coeff_d(1)*t^3 + coeff_d(2)*t^4 + coeff_d(3)*t^5;

        j_d = 6*coeff_d(1) + 24*coeff_d(2)*t + 60*coeff_d(3)*t^2;
        j_s = 6*coeff_s(1) + 24*coeff_s(2)*t;
        jerk_d = jerk_d + j_d^2;
        jerk_s = jerk_s + j_s^2;

        [xg, yg] = getCartesian(s_traj(i), d_traj(i), map_x, map_y, map_s);
        x_traj(i) = xg;
        y_traj(i) = yg;

        % 충돌 체크
        for j = 1:num_obs
            obs_dist = hypot(xg - obs_x(j), yg - obs_y(j));
            if obs_dist < (ego_radius + obs_r)
                is_collision = true;
            end
        end
    end

    x_all(:,k) = x_traj;
    y_all(:,k) = y_traj;

    if ~is_collision
        d_diff = (d_traj(end))^2;
        v_diff = (target_speed - (s_traj(end)-s_traj(1))/T)^2;
        cost_lat = K_J*jerk_d + K_T*T + K_D*d_diff;
        cost_lon = K_J*jerk_s + K_T*T + K_V*v_diff;
        costs(k) = K_LAT*cost_lat + K_LON*cost_lon;
    end

    trajectories{k,1} = x_traj;
    trajectories{k,2} = y_traj;
end

% === 유지 조건을 위한 persistent 변수들 ===
persistent prev_best_idx hold_count
if isempty(prev_best_idx)
    prev_best_idx = 2; % 초기엔 중앙 차선
    hold_count = 0;
end

% 최적 경로 선택
[best_cost, new_best_idx] = min(costs);

% 히스테리시스 조건
threshold = 5.0;                 % 얼마나 좋아야 바꿀지
hold_limit = 3.0 / dt;           % 유지 프레임 수 (3초)
current_cost = costs(prev_best_idx);

% 경로 변경 조건
if (new_best_idx ~= prev_best_idx) && ...
        (best_cost + threshold < current_cost || hold_count >= hold_limit)
    % 변경 허용
    prev_best_idx = new_best_idx;
    hold_count = 0;
else
    % 경로 유지
    new_best_idx = prev_best_idx;
    hold_count = hold_count + 1;
end

% 최종 선택
x_best = trajectories{new_best_idx,1};
y_best = trajectories{new_best_idx,2};

end

%% === 보조 함수 ===

function [s, d] = getFrenet(x, y, mapx, mapy, maps)
min_dist = inf; idx = 1;
for i = 1:length(mapx)-1
    dist = hypot(x - mapx(i), y - mapy(i));
    if dist < min_dist
        min_dist = dist;
        idx = i;
    end
end
dx = mapx(idx+1) - mapx(idx);
dy = mapy(idx+1) - mapy(idx);
seg_len = hypot(dx, dy);
proj = ((x - mapx(idx)) * dx + (y - mapy(idx)) * dy) / seg_len^2;
proj_x = mapx(idx) + proj * dx;
proj_y = mapy(idx) + proj * dy;
d = (x - proj_x) * (-dy/seg_len) + (y - proj_y) * (dx/seg_len);
s = maps(idx) + proj * seg_len;
end

function [x, y] = getCartesian(s, d, mapx, mapy, maps)
if s >= maps(end)
    s = maps(end) - 0.001;
end
idx_array = find(maps > s, 1);
if isempty(idx_array)
    idx = length(maps) - 1;
else
    idx = idx_array - 1;
end
if idx < 1
    idx = 1;
elseif idx >= length(mapx)
    idx = length(mapx) - 1;
end
mx0 = mapx(idx); mx1 = mapx(idx+1);
my0 = mapy(idx); my1 = mapy(idx+1);
dx_val = mx1 - mx0;
dy_val = my1 - my0;
heading = atan2(dy_val, dx_val);
ds = s - maps(idx);
base_x = mx0 + ds * cos(heading);
base_y = my0 + ds * sin(heading);
x = base_x - d * sin(heading);
y = base_y + d * cos(heading);
end

== matlab function Shin_com/Triggered Subsystem/MATLAB Function3 ==
  settings: sampleTime=0.05
  data: poly_coeff input; lateral_error output; velocity input; lookahead_time input; x_lookahead output
function [lateral_error, x_lookahead] = compute_lateral_error(poly_coeff, velocity, lookahead_time)
    % Lookahead 지점 계산
    x_lookahead = velocity * lookahead_time + 2.9;

    % 경로 상의 lookahead 지점에서의 y값 계산
    y_desired = polyval(poly_coeff, x_lookahead);

    % lateral error : 차량 y=0 위치와 경로 y_desired의 차이
    lateral_error = y_desired;
end
